simulink model "simpleDCMotor"  (R2025a)
settings: Solver=ode15s  StartTime=0.0  StopTime=30  RelTol=1e-3
undefined symbols (not defined in the file): b, J, K, L, R, V
settings Model: Creator=JPIRES3  LastModifiedBy=JPIRES3

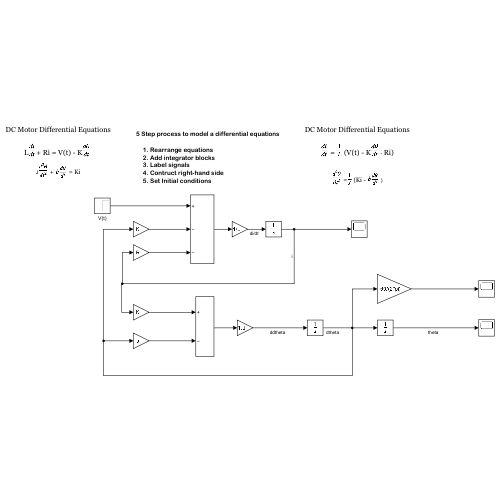
[thumbnail: Simulink's stored preview of the top-level diagram]
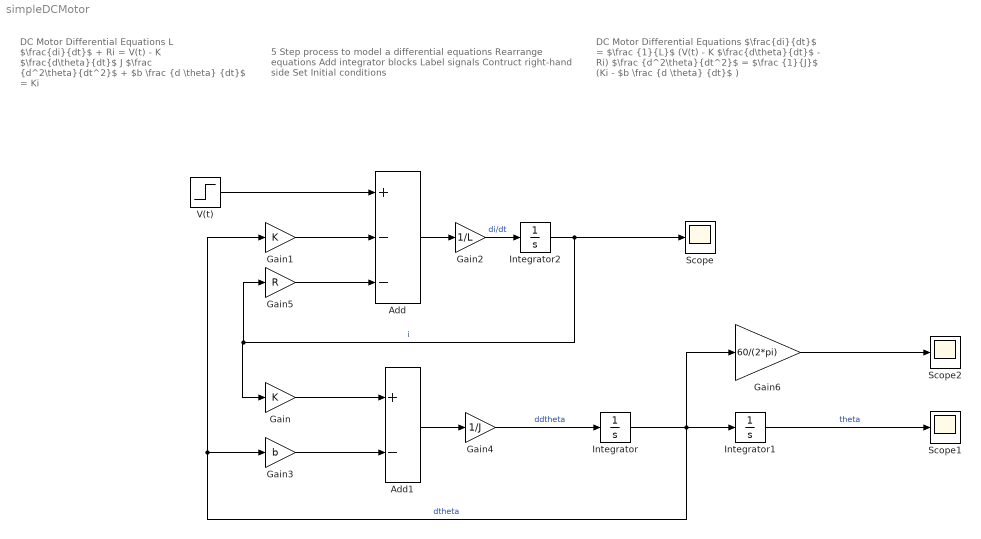
== system simpleDCMotor ==
  note: DC Motor Differential Equations
      |
      | L $\frac{di}{dt}$ + Ri = V(t) - K $\frac{d\theta}{dt}$
      | J $\frac {d^2\theta}{dt^2}$ + $b \frac {d \theta} {dt}$ = Ki
  note: 5 Step process to model a differential equations
      |
      | Rearrange equations
      | Add integrator blocks
      | Label signals
      | Contruct right-hand side
      | Set Initial conditions
  note: DC Motor Differential Equations
      |
      | $\frac{di}{dt}$ = $\frac {1}{L}$ (V(t) - K $\frac{d\theta}{dt}$ - Ri)
      |
      | $\frac {d^2\theta}{dt^2}$ = $\frac {1}{J}$ (Ki - $b \frac {d \theta} {dt}$ )
  Add : Sum  Inputs=+--
  Add1 : Sum  Inputs=+-
  Gain : Gain  Gain=K
  Gain1 : Gain  Gain=K
  Gain2 : Gain  Gain=1/L
  Gain3 : Gain  Gain=b
  Gain4 : Gain  Gain=1/J
  Gain5 : Gain  Gain=R
  Gain6 : Gain  Gain=60/(2*pi)
  Integrator : Integrator
  Integrator1 : Integrator
  Integrator2 : Integrator
  Scope : Scope
      settings: ActiveDisplayYMinimum=-0.027737152055078831  ActiveDisplayYMaximum=0.089409049553892117
  Scope1 : Scope
      settings: ActiveDisplayYMinimum=-0.14603038563974927  ActiveDisplayYMaximum=1.3142734707577437
  Scope2 : Scope
      settings: ActiveDisplayYMinimum=-1  ActiveDisplayYMaximum=1  DataLoggingVariableName=ScopeData2
  V(t) : Step  After=V  SampleTime=0
  wires:
  Add1/1 -> Gain4/1
  Integrator/1 -> Gain6/1, Integrator1/1, Gain1/1, Gain3/1  "dtheta"
  Integrator1/1 -> Scope1/1  "theta"
  Add/1 -> Gain2/1
  Integrator2/1 -> Scope/1, Gain5/1, Gain/1  "i"
  V(t)/1 -> Add/1
  Gain1/1 -> Add/2
  Gain2/1 -> Integrator2/1  "di/dt"
  Gain/1 -> Add1/1
  Gain3/1 -> Add1/2
  Gain4/1 -> Integrator/1  "ddtheta"
  Gain5/1 -> Add/3
  Gain6/1 -> Scope2/1
